simulink model "AERO60492_AMR_RigidBodyDynamics_2021"  (R2022a)
settings: Solver=VariableStepAuto  StartTime=0.0  StopTime=10.0  RelTol=1e-3
settings Model: Creator=z72217kw  LastModifiedBy=z72217kw
settings ModelReferenceCC: EnableRefExpFcnMdlSchedulingChecks=off
settings RTWCC: Description=Generic Real-Time Target

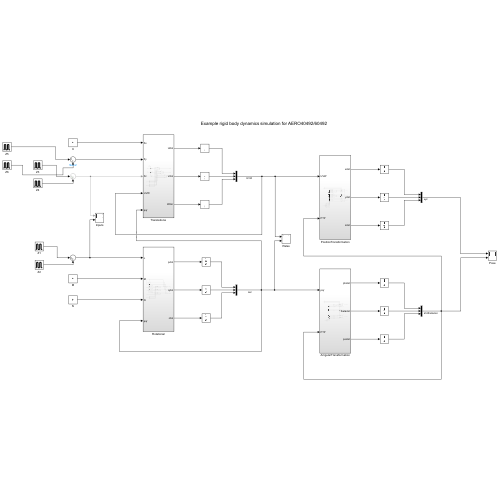
[thumbnail: Simulink's stored preview of the top-level diagram]
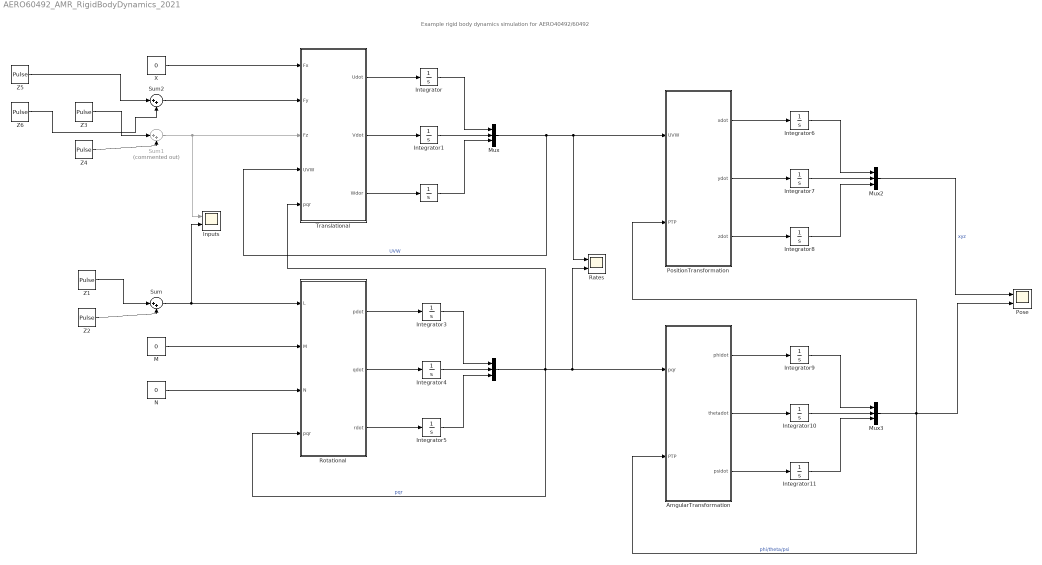
== system AERO60492_AMR_RigidBodyDynamics_2021 ==
  note: Example rigid body dynamics simulation for AERO40492/60492
  " " : Integrator
  "  " : Mux  Inputs=3
  AmgularTransformation : Subsystem
  Inputs : Scope  NumInputPorts=2
  Integrator{,1,3..11} (11 alike) : Integrator
  M : Constant  Value=0
  Mux : Mux  Inputs=3
  Mux2 : Mux  Inputs=3
  Mux3 : Mux  Inputs=3
  N : Constant  Value=0
  Pose : Scope  NumInputPorts=2
  PositionTransformation : Subsystem
  Rates : Scope  NumInputPorts=2
  Rotational : Subsystem
  Sum : Sum  Inputs=|++
  Sum1 : Sum  Commented=on  Inputs=|++
  Sum2 : Sum  Inputs=|++
  Translational : Subsystem
  X : Constant  Value=0
  Z1 : DiscretePulseGenerator  PulseType=Time based  Amplitude=-0.5  Period=100  PhaseDelay=4
  Z2 : DiscretePulseGenerator  PulseType=Time based  Amplitude=0.5  Period=100  PhaseDelay=5
  Z3 : DiscretePulseGenerator  PulseType=Time based  Period=100  PhaseDelay=1
  Z4 : DiscretePulseGenerator  PulseType=Time based  Amplitude=-1  Period=100  PhaseDelay=2
  Z5 : DiscretePulseGenerator  PulseType=Time based  Period=100  PhaseDelay=1
  Z6 : DiscretePulseGenerator  PulseType=Time based  Amplitude=-1  Period=100  PhaseDelay=2
  wires:
  X/1 -> Translational/1(Fx)
  Sum2/1 -> Translational/2(Fy)
  Sum1/1 -> Translational/3(Fz), Inputs/1
  M/1 -> Rotational/2(M)
  N/1 -> Rotational/3(N)
  Translational/1(Udot) -> Integrator/1
  Translational/3(Wdor) -> " "/1
  Translational/2(Vdot) -> Integrator1/1
  Rotational/1(pdot) -> Integrator3/1
  Rotational/2(qdot) -> Integrator4/1
  Rotational/3(rdot) -> Integrator5/1
  Integrator/1 -> Mux/1
  Integrator1/1 -> Mux/2
  " "/1 -> Mux/3
  Integrator3/1 -> "  "/1
  Integrator4/1 -> "  "/2
  Integrator5/1 -> "  "/3
  Mux/1 -> PositionTransformation/1(UVW), Rates/1, Translational/4(UVW)  "UVW"
  "  "/1 -> Translational/5(pqr), AmgularTransformation/1(pqr), Rates/2, Rotational/4(pqr)  "pqr"
  PositionTransformation/1(xdot) -> Integrator6/1
  PositionTransformation/2(ydot) -> Integrator7/1
  PositionTransformation/3(zdot) -> Integrator8/1
  AmgularTransformation/1(phidot) -> Integrator9/1
  AmgularTransformation/2(thetadot) -> Integrator10/1
  AmgularTransformation/3(psidot) -> Integrator11/1
  Integrator6/1 -> Mux2/1
  Integrator7/1 -> Mux2/2
  Integrator8/1 -> Mux2/3
  Integrator9/1 -> Mux3/1
  Integrator10/1 -> Mux3/2
  Integrator11/1 -> Mux3/3
  Mux2/1 -> Pose/1  "xyz"
  Mux3/1 -> PositionTransformation/2(PTP), Pose/2, AmgularTransformation/2(PTP)  "phi/theta/psi"
  Z1/1 -> Sum/1
  Z2/1 -> Sum/2
  Sum/1 -> Rotational/1(L), Inputs/2
  Z4/1 -> Sum1/2
  Z3/1 -> Sum1/1
  Z5/1 -> Sum2/1
  Z6/1 -> Sum2/2

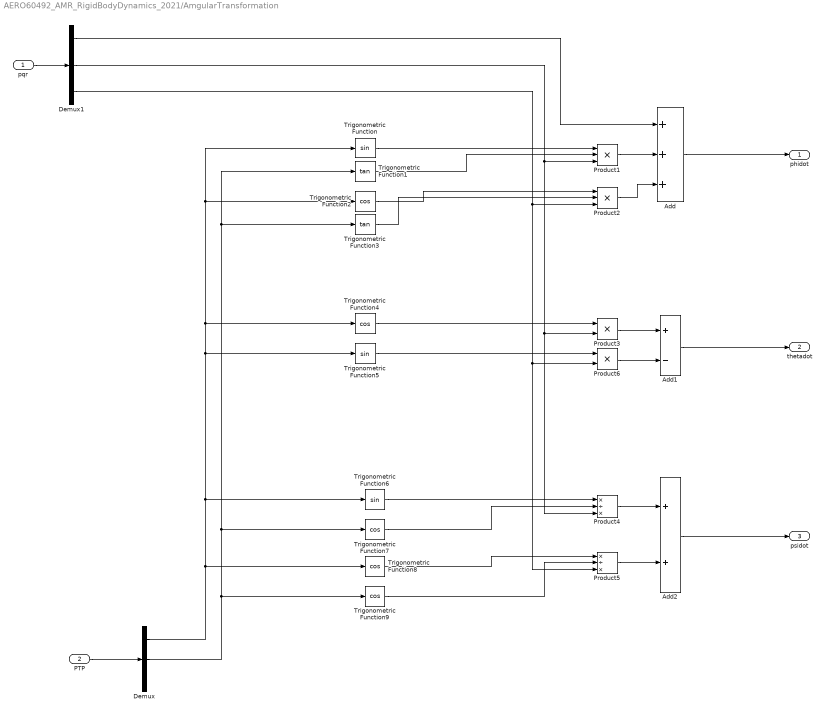
== system AERO60492_AMR_RigidBodyDynamics_2021/AmgularTransformation ==
  pqr : Inport
  PTP : Inport  Port=2
  Add : Sum  Inputs=+++
  Add1 : Sum  Inputs=+-
  Add2 : Sum
  Demux : Demux  Outputs=3
  Demux1 : Demux  Outputs=3
  Product1 : Product  Inputs=3
  Product2 : Product  Inputs=3
  Product3 : Product
  Product4 : Product  Inputs=*/*
  Product5 : Product  Inputs=*/*
  Product6 : Product
  Trigonometric Function : Trigonometry
  Trigonometric Function1 : Trigonometry  Operator=tan
  Trigonometric Function{2,4,7..9} (5 alike) : Trigonometry  Operator=cos
  Trigonometric Function3 : Trigonometry  Operator=tan
  Trigonometric Function5 : Trigonometry
  Trigonometric Function6 : Trigonometry
  phidot : Outport
  thetadot : Outport  Port=2
  psidot : Outport  Port=3
  wires:
  PTP/1 -> Demux/1
  Add/1 -> phidot/1
  Add2/1 -> psidot/1
  Add1/1 -> thetadot/1
  Demux1/1 -> Add/1
  Product1/1 -> Add/2
  Product2/1 -> Add/3
  Product3/1 -> Add1/1
  Product6/1 -> Add1/2
  Product4/1 -> Add2/1
  Product5/1 -> Add2/2
  Demux/1 -> Trigonometric Function6/1, Trigonometric Function2/1, Trigonometric Function/1, Trigonometric Function4/1, Trigonometric Function5/1, Trigonometric Function8/1
  Demux/2 -> Trigonometric Function3/1, Trigonometric Function1/1, Trigonometric Function7/1, Trigonometric Function9/1
  Trigonometric Function/1 -> Product1/1
  Trigonometric Function1/1 -> Product1/2
  Demux1/2 -> Product3/2, Product4/3, Product1/3
  Trigonometric Function2/1 -> Product2/1
  Trigonometric Function3/1 -> Product2/2
  Demux1/3 -> Product6/2, Product5/3, Product2/3
  Trigonometric Function4/1 -> Product3/1
  Trigonometric Function5/1 -> Product6/1
  Trigonometric Function6/1 -> Product4/1
  Trigonometric Function7/1 -> Product4/2
  Trigonometric Function8/1 -> Product5/1
  Trigonometric Function9/1 -> Product5/2
  pqr/1 -> Demux1/1

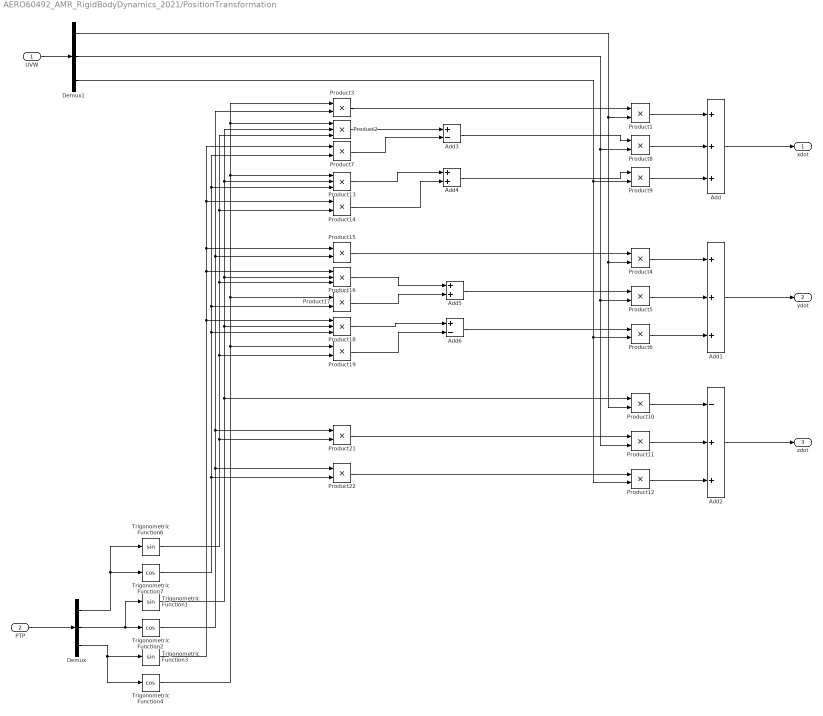
== system AERO60492_AMR_RigidBodyDynamics_2021/PositionTransformation ==
  UVW : Inport
  PTP : Inport  Port=2
  Add : Sum  Inputs=+++
  Add1 : Sum  Inputs=+++
  Add2 : Sum  Inputs=-++
  Add3 : Sum  Inputs=+-
  Add4 : Sum
  Add5 : Sum
  Add6 : Sum  Inputs=+-
  Demux : Demux  Outputs=3
  Demux1 : Demux  Outputs=3
  Product{1,3..12,14..15,17,19,21..22} (17 alike) : Product
  Product{2,13,16,18} (4 alike) : Product  Inputs=3
  Trigonometric Function1 : Trigonometry
  Trigonometric Function2 : Trigonometry  Operator=cos
  Trigonometric Function3 : Trigonometry
  Trigonometric Function4 : Trigonometry  Operator=cos
  Trigonometric Function6 : Trigonometry
  Trigonometric Function7 : Trigonometry  Operator=cos
  xdot : Outport
  ydot : Outport  Port=2
  zdot : Outport  Port=3
  wires:
  UVW/1 -> Demux1/1
  Add1/1 -> ydot/1
  Add2/1 -> zdot/1
  Add/1 -> xdot/1
  PTP/1 -> Demux/1
  Demux/1 -> Trigonometric Function6/1, Trigonometric Function7/1
  Demux/2 -> Trigonometric Function2/1, Trigonometric Function1/1
  Demux/3 -> Trigonometric Function4/1, Trigonometric Function3/1
  Trigonometric Function4/1 -> Product13/1, Product3/1, Product2/1, Product17/1, Product19/1
  Trigonometric Function2/1 -> Product15/2, Product3/2, Product21/1, Product22/1
  Product3/1 -> Product1/1
  Demux1/1 -> Product10/2, Product4/2, Product1/2
  Product1/1 -> Add/1
  Trigonometric Function6/1 -> Product21/2, Product19/2, Product16/3, Product2/3, Product14/2
  Trigonometric Function3/1 -> Product16/1, Product14/1, Product7/1, Product15/1, Product18/1
  Trigonometric Function7/1 -> Product18/3, Product13/3, Product7/2, Product17/2, Product22/2
  Product2/1 -> Add3/1
  Product7/1 -> Add3/2
  Add3/1 -> Product8/1
  Demux1/2 -> Product11/2, Product5/2, Product8/2
  Product8/1 -> Add/2
  Product9/1 -> Add/3
  Demux1/3 -> Product12/2, Product6/2, Product9/2
  Product4/1 -> Add1/1
  Product5/1 -> Add1/2
  Product6/1 -> Add1/3
  Product10/1 -> Add2/1
  Product11/1 -> Add2/2
  Product12/1 -> Add2/3
  Add4/1 -> Product9/1
  Product13/1 -> Add4/1
  Product14/1 -> Add4/2
  Product15/1 -> Product4/1
  Add5/1 -> Product5/1
  Product16/1 -> Add5/1
  Product17/1 -> Add5/2
  Add6/1 -> Product6/1
  Product18/1 -> Add6/1
  Product19/1 -> Add6/2
  Trigonometric Function1/1 -> Product18/2, Product16/2, Product13/2, Product2/2, Product10/1
  Product21/1 -> Product11/1
  Product22/1 -> Product12/1

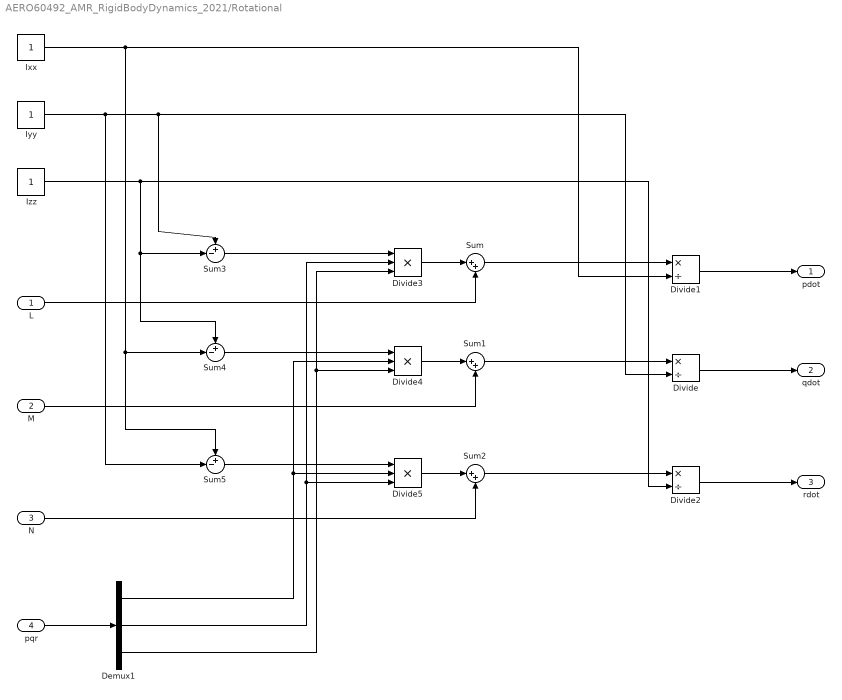
== system AERO60492_AMR_RigidBodyDynamics_2021/Rotational ==
  L : Inport
  M : Inport  Port=2
  N : Inport  Port=3
  pqr : Inport  Port=4
  Demux1 : Demux  Outputs=3
  Divide : Product  Inputs=*/
  Divide1 : Product  Inputs=*/
  Divide2 : Product  Inputs=*/
  Divide3 : Product  Inputs=***
  Divide4 : Product  Inputs=***
  Divide5 : Product  Inputs=***
  Ixx : Constant
  Iyy : Constant
  Izz : Constant
  Sum : Sum  Inputs=|++
  Sum1 : Sum  Inputs=|++
  Sum2 : Sum  Inputs=|++
  Sum3 : Sum  Inputs=+-|
  Sum4 : Sum  Inputs=+-|
  Sum5 : Sum  Inputs=+-|
  pdot : Outport
  qdot : Outport  Port=2
  rdot : Outport  Port=3
  wires:
  pqr/1 -> Demux1/1
  Ixx/1 -> Sum5/1, Sum4/2, Divide1/2
  Iyy/1 -> Sum5/2, Divide/2, Sum3/1
  Izz/1 -> Divide2/2, Sum3/2, Sum4/1
  Divide1/1 -> pdot/1
  Divide/1 -> qdot/1
  Divide2/1 -> rdot/1
  Demux1/2 -> Divide5/3, Divide3/2
  Demux1/3 -> Divide3/3, Divide4/3
  Demux1/1 -> Divide5/2, Divide4/2
  L/1 -> Sum/2
  M/1 -> Sum1/2
  N/1 -> Sum2/2
  Divide3/1 -> Sum/1
  Divide4/1 -> Sum1/1
  Divide5/1 -> Sum2/1
  Sum2/1 -> Divide2/1
  Sum1/1 -> Divide/1
  Sum/1 -> Divide1/1
  Sum3/1 -> Divide3/1
  Sum4/1 -> Divide4/1
  Sum5/1 -> Divide5/1

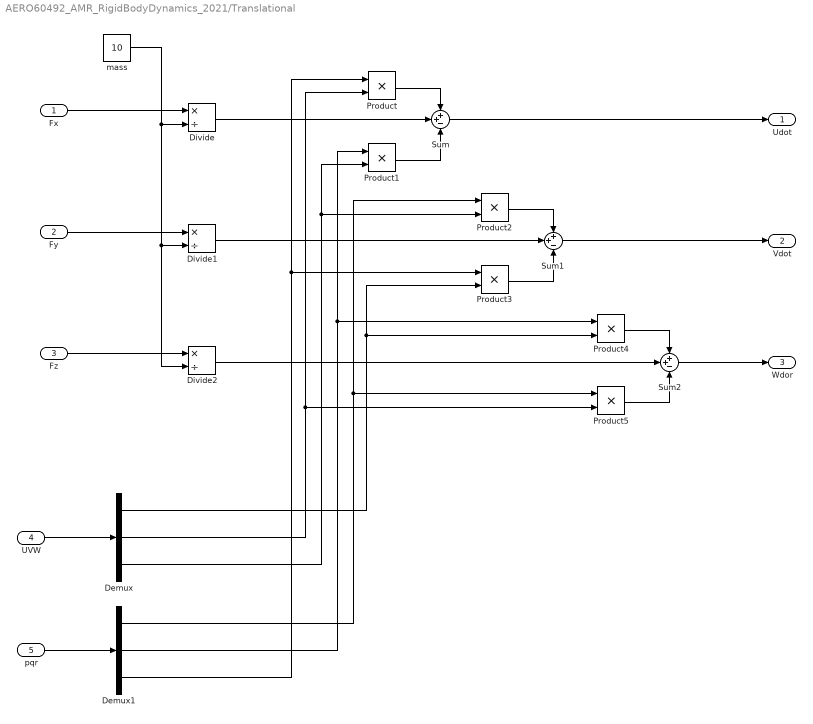
== system AERO60492_AMR_RigidBodyDynamics_2021/Translational ==
  Fx : Inport
  Fy : Inport  Port=2
  Fz : Inport  Port=3
  UVW : Inport  Port=4
  pqr : Inport  Port=5
  Demux : Demux  Outputs=3
  Demux1 : Demux  Outputs=3
  Divide : Product  Inputs=*/
  Divide1 : Product  Inputs=*/
  Divide2 : Product  Inputs=*/
  Product{,1..5} (6 alike) : Product
  Sum : Sum  Inputs=++-
  Sum1 : Sum  Inputs=++-
  Sum2 : Sum  Inputs=++-
  mass : Constant  Value=10
  Udot : Outport
  Vdot : Outport  Port=2
  Wdor : Outport  Port=3
  wires:
  mass/1 -> Divide2/2, Divide1/2, Divide/2
  Fx/1 -> Divide/1
  Fy/1 -> Divide1/1
  Fz/1 -> Divide2/1
  UVW/1 -> Demux/1
  pqr/1 -> Demux1/1
  Divide/1 -> Sum/2
  Product1/1 -> Sum/3
  Product/1 -> Sum/1
  Product3/1 -> Sum1/3
  Product2/1 -> Sum1/1
  Divide1/1 -> Sum1/2
  Sum1/1 -> Vdot/1
  Sum/1 -> Udot/1
  Product5/1 -> Sum2/3
  Product4/1 -> Sum2/1
  Divide2/1 -> Sum2/2
  Sum2/1 -> Wdor/1
  Demux1/3 -> Product/1, Product3/1
  Demux/2 -> Product5/2, Product/2
  Demux1/2 -> Product1/1, Product4/1
  Demux1/1 -> Product5/1, Product2/1
  Demux/3 -> Product2/2, Product1/2
  Demux/1 -> Product4/2, Product3/2
